simulink model "IMC_Controller"  (R2019b)
settings: Solver=VariableStepAuto  StartTime=0.0  StopTime=10.0  RelTol=1e-3
PostLoadFcn:
  | if any(exist('dsrtsu_mdlpostloadfcn', 'file') ~= 0), dsrtsu_mdlpostloadfcn('Execute', bdroot); end
undefined symbols (not defined in the file): I, P
libraries: simulink x6
settings Model: DSRTSU_INTERNAL_RTI_VER=550  DSRTSU_INTERNAL_RTI_TYPE=rti1104  RTICANMMDATA=struct('GeneralSetupData',struct('modelroot',['G:\RemoteLabs\RL git repos\Three Tank System set-up\dynamics-and-process-control-6e8x0\Teacher_files'],'generalsettings',struct('filesettings',struct('destfolder',struct('Name','RTICANMM_FILES','Check',1),'buildfolder',struct('Name','.','Check',1),'AbsDestfolder',struct('Name',['G:\RemoteLabs\RL git repos\Three Tank System set-up\dynamics-and-process-control-6e8x0\Teacher_files\RTICANMM_FILES']),'AbsBuildfolder',struct('Name',['G:\RemoteLabs\RL git repos\Three Tank System set-up\dynamics-and-process-control-6e8x0\Teacher_files']))),'options',struct('addpaths',1,'rmpaths',1,'addtrcexclusion',true,'cannavigator',struct('checkmonitoring',0),'show_usrtrc',0,'use_usrtrc',0),'advanced',struct('options',ones(1,100)),'MPSetup',{{}},'RTI',struct('Type','GRT','Ver','','Date',''),'modelname','RL_TTS1_Controller','block','RL_TTS1_Controller'))  DSRTSU_INTERNAL_RTIFPGA=150  Creator=whendrix  LastModifiedBy=20191255
settings SFSimCC: CustomCodeUndefinedFunction=UseInterfaceOnly

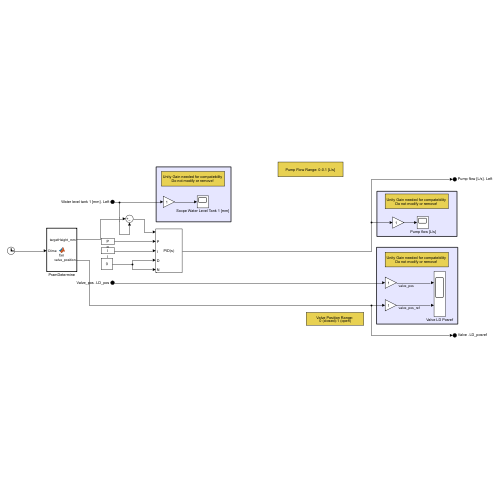
[thumbnail: Simulink's stored preview of the top-level diagram]
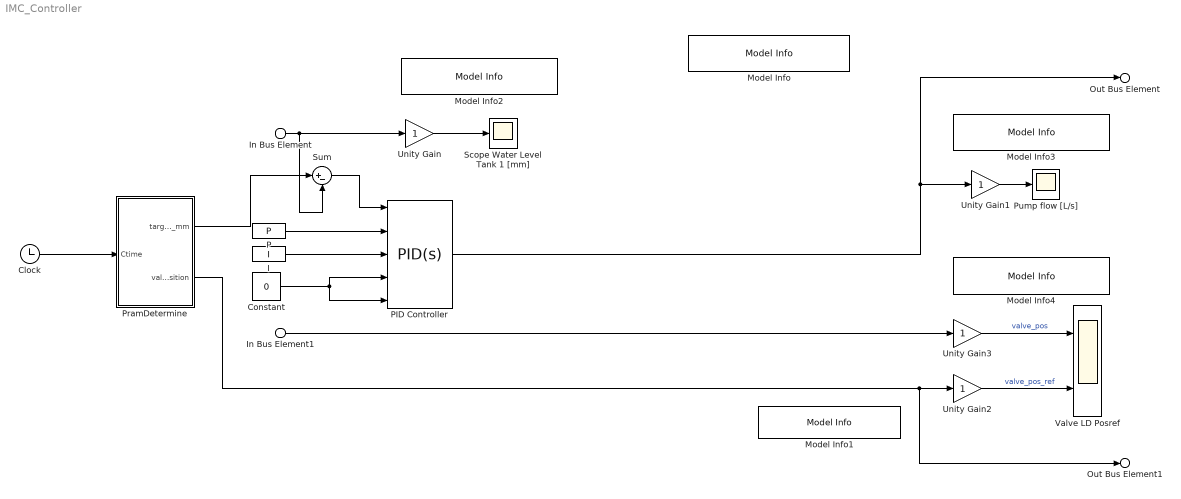
== system IMC_Controller ==
  In Bus Element : Inport  PortName=Water level tank 1 [mm]  Element=Left
  In Bus Element1 : Inport  Port=2  PortName=Valve_pos  Element=LD_pos
  " Pump flow [L/s]" : Scope
  Clock : Clock
  Constant : Constant  Value=0
  I : Constant  Value=I
  Model Info : simulink/Model-Wide Utilities/Model Info  Frame=on  DisplayStringWithTags=Pump Flow Range: 0-0.1 [L/s]  HorizontalTextAlignment=Center  LeftAlignmentValue=0.5
  Model Info1 : simulink/Model-Wide Utilities/Model Info  Frame=on  DisplayStringWithTags=|  HorizontalTextAlignment=Center  LeftAlignmentValue=0.5
      | Valve Position Range:
      |  0 (closed)-1 (open)
  Model Info2 : simulink/Model-Wide Utilities/Model Info  Frame=on  DisplayStringWithTags=Unity Gain needed for compatebility Do not modify or remove!  HorizontalTextAlignment=Center  LeftAlignmentValue=0.5
  Model Info3 : simulink/Model-Wide Utilities/Model Info  Frame=on  DisplayStringWithTags=Unity Gain needed for compatebility Do not modify or remove!  HorizontalTextAlignment=Center  LeftAlignmentValue=0.5
  Model Info4 : simulink/Model-Wide Utilities/Model Info  Frame=on  DisplayStringWithTags=Unity Gain needed for compatebility Do not modify or remove!  HorizontalTextAlignment=Center  LeftAlignmentValue=0.5
  P : Constant  Value=P
  PID Controller : simulink/Continuous/PID Controller  Controller=PID  Form=Parallel  TimeDomain=Continuous-time  SampleTime=-1  IntegratorMethod=Forward Euler  FilterMethod=Forward Euler  ControllerParametersSource=external  P=1  I=1  D=0  UseFilter=on  N=100  TunerSelectOption=Transfer Function Based (PID Tuner App)  InitialConditionSource=internal  InitialConditionForIntegrator=0  InitialConditionForFilter=0  DifferentiatorICPrevScaledInput=0  ExternalReset=none  TrackingMode=off  Kt=1  LimitOutput=off  UpperSaturationLimit=inf  LowerSaturationLimit=-inf  LinearizeAsGain=on  AntiWindupMode=none  Kb=1  POutMin=[]  POutMax=[]  IOutMin=[]  IOutMax=[]  DOutMin=[]  DOutMax=[]  NOutMin=[]  NOutMax=[]  SumOutMin=[]  SumOutMax=[]  SaturationOutMin=[]  SaturationOutMax=[]  PParamMin=[]  PParamMax=[]  IParamMin=[]  IParamMax=[]  DParamMin=[]  DParamMax=[]  NParamMin=[]  NParamMax=[]  KbParamMin=[]  KbParamMax=[]  KtParamMin=[]  KtParamMax=[]  KbOutMin=[]  KbOutMax=[]  KtOutMin=[]  KtOutMax=[]  IntegratorOutMin=[]  IntegratorOutMax=[]  FilterOutMin=[]  FilterOutMax=[]  SumI1OutMin=[]  SumI1OutMax=[]  SumI2OutMin=[]  SumI2OutMax=[]  SumI3OutMin=[]  SumI3OutMax=[]  SumI4OutMin=[]  SumI4OutMax=[]  SumDOutMin=[]  SumDOutMax=[]  DifferentiatorOutMin=[]  DifferentiatorOutMax=[]  FilterDiffOutCoefMin=[]  FilterDiffOutCoefMax=[]  ReciprocalOutMin=[]  ReciprocalOutMax=[]  SumDenOutMin=[]  SumDenOutMax=[]  SumNumOutMin=[]  SumNumOutMax=[]  DivideOutMin=[]  DivideOutMax=[]  IntegratorContinuousStateAttributes=''  IntegratorStateMustResolveToSignalObject=off  IntegratorRTWStateStorageClass=Auto  FilterContinuousStateAttributes=''  FilterStateMustResolveToSignalObject=off  FilterRTWStateStorageClass=Auto  ParallelPVariant=ExternalParameters  IdealPVariant=Disabled  IVariant=ExternalParameters  DVariant=ExternalParameters  IntegratorVariant=Continuous  SatVariant=Disabled  AWVariant=Passthrough  PCopyVariant=Disabled  TRVariant=Disabled  FdbkBlocksVariant=Forward  IdealPFdbkVariant=Disabled  SatFdbkVariant=Disabled  DerivativeFilterVariant=ContFilter  NVariant=ExternalParameters  NCopyVariant=Disabled  FilterICVariant=InternalICsFilter  IntegratorICVariant=InternalICs  ExternalResetVariant=Disabled  TRSumVariant=Passthrough  SumFdbkVariant=Disabled  SumVariant=Sum_PID
  PramDetermine : MATLAB Function  TreatAsAtomicUnit=on
  Scope Water Level Tank 1 [mm] : Scope
  Sum : Sum  Inputs=|+-
  Unity Gain{,1..3} (4 alike) : Gain
  Valve LD Posref : Scope  NumInputPorts=2
  Out Bus Element : Outport  PortName=Pump flow [L/s]  Element=Left
  Out Bus Element1 : Outport  Port=2  PortName=Valve  Element=LD_posref
  wires:
  In Bus Element/1 -> Unity Gain/1, Sum/2
  Unity Gain/1 -> Scope Water Level Tank 1 [mm]/1
  Unity Gain1/1 -> " Pump flow [L/s]"/1
  Unity Gain3/1 -> Valve LD Posref/1  "valve_pos"
  In Bus Element1/1 -> Unity Gain3/1
  Unity Gain2/1 -> Valve LD Posref/2  "valve_pos_ref"
  PramDetermine/1(targetHeight_mm) -> Sum/1
  Sum/1 -> PID Controller/1
  P/1 -> PID Controller/2
  I/1 -> PID Controller/3
  Constant/1 -> PID Controller/5, PID Controller/4
  PID Controller/1 -> Out Bus Element/1, Unity Gain1/1
  PramDetermine/2(valve_position) -> Out Bus Element1/1, Unity Gain2/1
  Clock/1 -> PramDetermine/1(Ctime)

== matlab function IMC_Controller/PramDetermine ==
  data: Ctime input; targetHeight_mm output; valve_position output
function [targetHeight_mm, valve_position] = fxn(Ctime)

[targetHeight_mm, valve_position] = PramDetermine(Ctime);

end
